simulink library "csc_thl_thrusters_lander_lib"  (R2015b)
settings: Solver=ode45  StartTime=0.0  StopTime=10.0  RelTol=1e-3
undefined symbols (not defined in the file or in its folder): mpl_gn2_mass_initial, mpl_htp_mass_initial, mpl_rp1_mass_initial
libraries: simulink x6, util_info_lib x1, csc_tdl_thruster_dynamics_collection_lib x1, csu_tfl_thruster_forces_lander_lib_diag x1, csu_tpl_thruster_propellant_lander_lib x1
settings Model: Creator=Mark Agbayani  LastModifiedBy=jimkaidy
settings DataIOCC: SaveFormat=Array
settings DebuggingCC: SolverPrmCheckMsg=warning
settings HardwareCC: ProdBitPerPointer=32  ProdLargestAtomicFloat=None  ProdIntDivRoundTo=Undefined  ProdEndianess=Unspecified  ProdWordSize=32  ProdHWDeviceType=32-bit Generic
settings GRTTargetCC: GeneratePreprocessorConditionals=Disable all
settings ConfigComp: CovModelRefEnable=Off  CovSFcnEnable=off

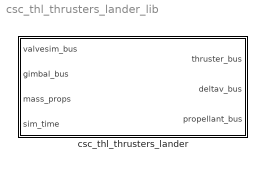
== system csc_thl_thrusters_lander_lib ==
  csc_thl_thrusters_lander : Subsystem

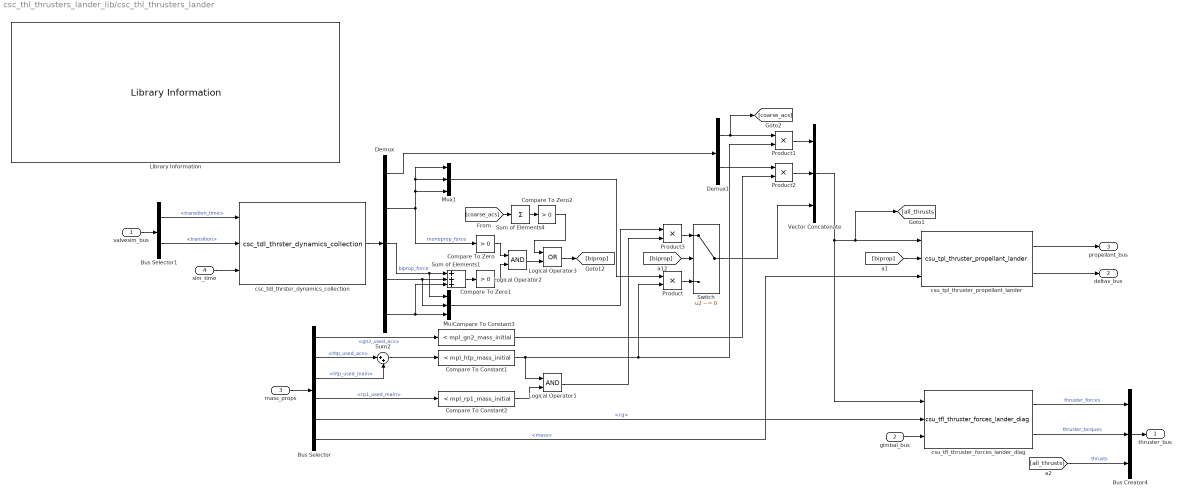
== system csc_thl_thrusters_lander_lib/csc_thl_thrusters_lander ==
  valvesim_bus : Inport
  gimbal_bus : Inport  Port=2
  mass_props : Inport  Port=3
  sim_time : Inport  Port=4
  Bus Creator4 : BusCreator  Inputs=3  OutDataTypeStr=Bus: actuator_msg_t
  Bus Selector : BusSelector  OutputSignals=gn2_used_acs,htp_used_acs,htp_used_main,rp1_used_main,cg,mass
  Bus Selector1 : BusSelector  OutputSignals=transition_time,transition
  Compare To Constant1 : simulink/Logic and Bit Operations/Compare To Constant  relop=<  const=mpl_htp_mass_initial  OutDataTypeStr=uint8
  Compare To Constant2 : simulink/Logic and Bit Operations/Compare To Constant  relop=<  const=mpl_rp1_mass_initial  OutDataTypeStr=uint8
  Compare To Constant3 : simulink/Logic and Bit Operations/Compare To Constant  relop=<  const=mpl_gn2_mass_initial  OutDataTypeStr=uint8
  Compare To Zero : simulink/Logic and Bit Operations/Compare To Zero  relop=>  OutDataTypeStr=boolean
  Compare To Zero1 : simulink/Logic and Bit Operations/Compare To Zero  relop=>  OutDataTypeStr=boolean
  Compare To Zero2 : simulink/Logic and Bit Operations/Compare To Zero  relop=>  OutDataTypeStr=boolean
  Demux : Demux  Outputs=[24 1 1 1 1]
  Demux1 : Demux  Outputs=[12 12]
  Library Information : util_info_lib/Library Information  owner='NONE'
  Logical Operator1 : Logic  AllPortsSameDT=off  OutDataTypeStr=boolean
  Logical Operator2 : Logic  AllPortsSameDT=off  OutDataTypeStr=boolean
  Logical Operator3 : Logic  Operator=OR  AllPortsSameDT=off  OutDataTypeStr=boolean
  Mux : Mux  Inputs=3
  Mux1 : Mux  Inputs=3
  Product{,1..3} (4 alike) : Product
  Sum of Elements1 : Sum  Inputs=+++
  Sum of Elements4 : Sum  Inputs=+
  Sum2 : Sum  Inputs=|++
  Switch : Switch  Criteria=u2 ~= 0
  Vector Concatenate : Concatenate  NumInputs=3
  csc_tdl_thrster_dynamics_collection : csc_tdl_thruster_dynamics_collection_lib/csc_tdl_thrster_dynamics_collection  SystemSampleTime=-1
  csu_tfl_thruster_forces_lander_diag : csu_tfl_thruster_forces_lander_lib_diag/csu_tfl_thruster_forces_lander_diag
  csu_tpl_thruster_propellant_lander : csu_tpl_thruster_propellant_lander_lib/csu_tpl_thruster_propellant_lander
  thruster_bus : Outport
  deltav_bus : Outport  Port=2
  propellant_bus : Outport  Port=3
  wires:
  gimbal_bus/1 -> csu_tfl_thruster_forces_lander_diag/3
  Vector Concatenate/1 -> csu_tfl_thruster_forces_lander_diag/1, csu_tpl_thruster_propellant_lander/1, [all_thrusts]
  mass_props/1 -> Bus Selector/1
  Bus Selector/6 -> csu_tpl_thruster_propellant_lander/3  "<mass>"
  Bus Selector/5 -> csu_tfl_thruster_forces_lander_diag/2  "<cg>"
  sim_time/1 -> csc_tdl_thrster_dynamics_collection/3
  valvesim_bus/1 -> Bus Selector1/1
  csc_tdl_thrster_dynamics_collection/1 -> Demux/1
  Demux/2 -> Compare To Zero/1, Mux1/3, Mux1/2, Mux1/1  "monoprop_force"
  Demux/1 -> Demux1/1
  csu_tpl_thruster_propellant_lander/2 -> deltav_bus/1
  csu_tpl_thruster_propellant_lander/1 -> propellant_bus/1
  [biprop] -> Switch/2
  [biprop] -> csu_tpl_thruster_propellant_lander/2
  Bus Selector1/2 -> csc_tdl_thrster_dynamics_collection/2  "<transition>"
  Bus Selector1/1 -> csc_tdl_thrster_dynamics_collection/1  "<transition_time>"
  Bus Creator4/1 -> thruster_bus/1
  csu_tfl_thruster_forces_lander_diag/2 -> Bus Creator4/2  "thruster_torques"
  csu_tfl_thruster_forces_lander_diag/1 -> Bus Creator4/1  "thruster_forces"
  Compare To Zero/1 -> Logical Operator2/1
  Compare To Zero1/1 -> Logical Operator2/2
  [all_thrusts] -> Bus Creator4/3  "thrusts"
  Bus Selector/1 -> Compare To Constant3/1  "<gn2_used_acs>"
  Bus Selector/4 -> Compare To Constant2/1  "<rp1_used_main>"
  Sum2/1 -> Compare To Constant1/1
  Bus Selector/2 -> Sum2/1  "<htp_used_acs>"
  Bus Selector/3 -> Sum2/2  "<htp_used_main>"
  Demux1/1 -> [coarse_acs], Product1/1
  Demux1/2 -> Product2/1
  Product1/1 -> Vector Concatenate/1
  Product2/1 -> Vector Concatenate/2
  Switch/1 -> Vector Concatenate/3
  Compare To Constant3/1 -> Product2/2
  Compare To Constant2/1 -> Logical Operator1/2
  Product/1 -> Switch/3
  Compare To Constant1/1 -> Logical Operator1/1, Product/2, Product1/2
  Product3/1 -> Switch/1
  Logical Operator1/1 -> Product3/2
  Compare To Zero2/1 -> Logical Operator3/1
  [coarse_acs] -> Sum of Elements4/1
  Sum of Elements4/1 -> Compare To Zero2/1
  Logical Operator3/1 -> [biprop]
  Logical Operator2/1 -> Logical Operator3/2
  Sum of Elements1/1 -> Compare To Zero1/1
  Demux/3 -> Mux/1, Sum of Elements1/1  "biprop_force"
  Demux/4 -> Sum of Elements1/2, Mux/2
  Demux/5 -> Mux/3, Sum of Elements1/3
  Mux/1 -> Product3/1
  Mux1/1 -> Product/1
